simulink model "windrad"  (R2020a)
settings: Solver=ode45  StartTime=0.0  StopTime=20  FixedStep=1e-4  RelTol=1e-9
values from neighbouring files (symbols this model uses):
  a = 0.0158    [windrad_init.m]
  b = 0.00084    [windrad_init.m]
  Kp = b/a    (= 0.053164556962)    [windrad_init.m]
  T1 = 1/a    (= 63.2911392405)    [windrad_init.m]
  Tt = 0.2    [windrad_init.m]
undefined symbols (not defined in the file or in its folder): d
settings Model: Creator=seife  LastModifiedBy=Ravi Plenzdorf
settings DataIOCC: ReturnWorkspaceOutputs=off

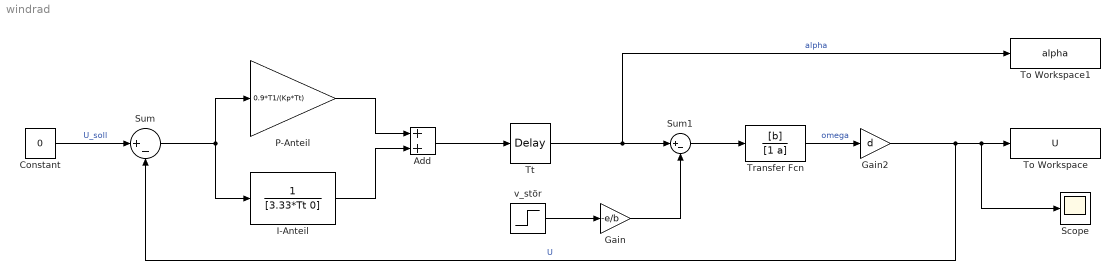
== system windrad ==
  Add : Sum
  Constant : Constant  Value=0
  Gain : Gain  Gain=-e/b
  Gain2 : Gain  Gain=d
  I-Anteil : TransferFcn  Denominator=[3.33*Tt 0]
  P-Anteil : Gain  Gain=0.9*T1/(Kp*Tt)
  Scope : Scope
  Sum : Sum  Inputs=|+-
  Sum1 : Sum  Inputs=|+-
  To Workspace : ToWorkspace  VariableName=U  SaveFormat=Timeseries  SampleTime=-1
  To Workspace1 : ToWorkspace  VariableName=alpha  SaveFormat=Timeseries  SampleTime=-1
  Transfer Fcn : TransferFcn  Numerator=[b]  Denominator=[1 a]
  Tt : TransportDelay  DelayTime=Tt
  v_stör : Step  Time=2  SampleTime=0
  wires:
  Constant/1 -> Sum/1  "U_soll"
  Tt/1 -> To Workspace1/1, Sum1/1  "alpha"
  Sum1/1 -> Transfer Fcn/1
  v_stör/1 -> Gain/1
  Gain/1 -> Sum1/2
  Gain2/1 -> Sum/2, Scope/1, To Workspace/1  "U"
  Transfer Fcn/1 -> Gain2/1  "omega"
  P-Anteil/1 -> Add/1
  I-Anteil/1 -> Add/2
  Sum/1 -> P-Anteil/1, I-Anteil/1
  Add/1 -> Tt/1
